simulink model "Two_compartment_TOP"  (R2019b)
settings: Solver=VariableStepAuto  StartTime=0.0  StopTime=time  RelTol=1e-3
values from neighbouring files (symbols this model uses):
  breath = 60/f    (= 4)    [Model_simulation.m]
  E1 = 10    [Model_simulation.m]
  E2 = 10    [Model_simulation.m]
  E_high = 100    [Model_simulation.m]
  E_th = 15    [Model_simulation.m]
  insptime = (ieratio(1)/(ieratio(1)+ieratio(2)))*100    [Model_simulation.m]
  Pcontrol = 5    [Model_simulation.m]
  PEEP = 5    [Model_simulation.m]
  R = 30    [Model_simulation.m]
  R1 = 5    [Model_simulation.m]
  TOP2 = 20    [Model_simulation.m]
  V0 = 2    [Model_simulation.m]
  V0_th = 4.6    [Model_simulation.m]
undefined symbols (not defined in the file or in its folder): TOP
settings Model: Creator=Amne  LastModifiedBy=Amne
settings DataIOCC: ReturnWorkspaceOutputs=off
settings DebuggingCC: ArithmeticOperatorsInVariantConditions=warning
settings SFSimCC: SimUseLocalCustomCode=off  CustomCodeUndefinedFunction=UseInterfaceOnly
settings RTWCC: RTWUseLocalCustomCode=off

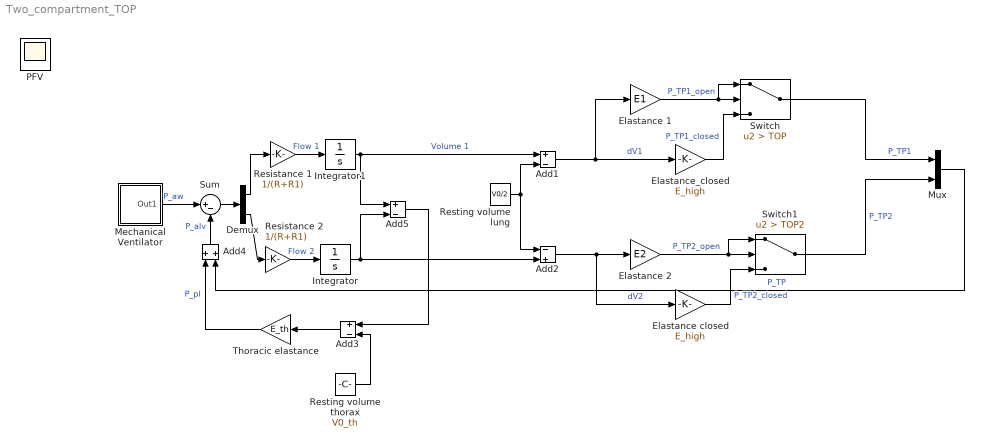
== system Two_compartment_TOP ==
  Add1 : Sum  Inputs=+-
  Add2 : Sum  Inputs=-+
  Add3 : Sum  Inputs=+-
  Add4 : Sum
  Add5 : Sum  Inputs=+-
  Demux : Demux  Outputs=2
  Elastance 1 : Gain  Gain=E1
  "Elastance 2 " : Gain  Gain=E2
  Elastance closed : Gain  Gain=E_high
  Elastance_closed : Gain  Gain=E_high
  Integrator : Integrator
  Integrator1 : Integrator
  "Mechanical Ventilator " : Subsystem
  Mux : Mux  Inputs=2
  Resistance 1 : Gain  Gain=1/(R+R1)
  Resistance 2 : Gain  Gain=1/(R+R1)
  "Resting volume lung " : Constant  Value=V0/2
  Resting volume thorax : Constant  Value=V0_th
  Sum : Sum  Inputs=|+-
  Switch : Switch  Criteria=u2 > Threshold  Threshold=TOP
  Switch1 : Switch  Criteria=u2 > Threshold  Threshold=TOP2
  Thoracic elastance : Gain  Gain=E_th
  PFV : Scope
  wires:
  "Mechanical Ventilator "/1(Out1) -> Sum/1  "P_aw"
  Resistance 1/1 -> Integrator1/1  "Flow 1"
  Elastance 1/1 -> Switch/1, Switch/2  "P_TP1_open"
  Mux/1 -> Add4/2  "P_TP"
  Add2/1 -> "Elastance 2 "/1, Elastance closed/1  "dV2"
  Add1/1 -> Elastance 1/1, Elastance_closed/1  "dV1"
  Resting volume thorax/1 -> Add3/2
  Add3/1 -> Thoracic elastance/1
  Thoracic elastance/1 -> Add4/1  "P_pl"
  Add4/1 -> Sum/2  "P_alv"
  "Resting volume lung "/1 -> Add2/1, Add1/2
  Elastance_closed/1 -> Switch/3  "P_TP1_closed"
  Switch/1 -> Mux/1  "P_TP1"
  "Elastance 2 "/1 -> Switch1/2, Switch1/1  "P_TP2_open"
  Switch1/1 -> Mux/2  "P_TP2"
  Elastance closed/1 -> Switch1/3  "P_TP2_closed"
  Integrator/1 -> Add5/2, Add2/2
  Sum/1 -> Demux/1
  Demux/1 -> Resistance 1/1
  Demux/2 -> Resistance 2/1
  Resistance 2/1 -> Integrator/1  "Flow 2"
  Integrator1/1 -> Add5/1, Add1/1  "Volume 1"
  Add5/1 -> Add3/1

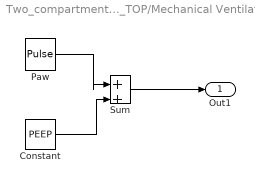
== system Two_compartment_TOP/Mechanical Ventilator  ==
  Constant : Constant  Value=PEEP  SampleTime=0.1
  Paw : DiscretePulseGenerator  PulseType=Time based  Amplitude=Pcontrol  Period=breath  PulseWidth=insptime  PhaseDelay=2  SampleTime=0.1
  Sum : Sum  Inputs=|++
  Out1 : Outport  VectorParamsAs1DForOutWhenUnconnected=off
  wires:
  Paw/1 -> Sum/1
  Constant/1 -> Sum/2
  Sum/1 -> Out1/1
